simulink subsystem "US_016"  (R2023b)
settings: Solver=VariableStepAuto  StartTime=0.0  StopTime=10.0  RelTol=1e-3
libraries: arduinolib x2
settings Model: Creator=javie  LastModifiedBy=javie

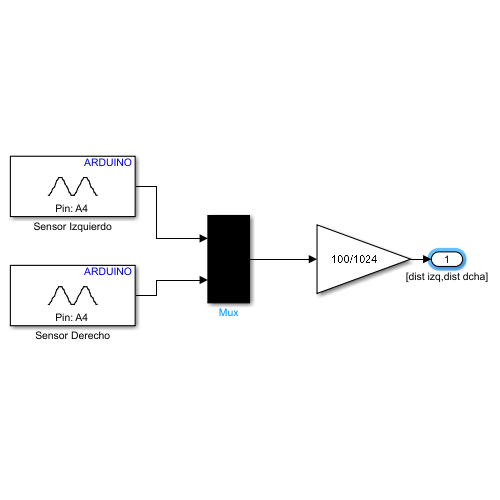
[thumbnail: Simulink's stored preview of the top-level diagram]
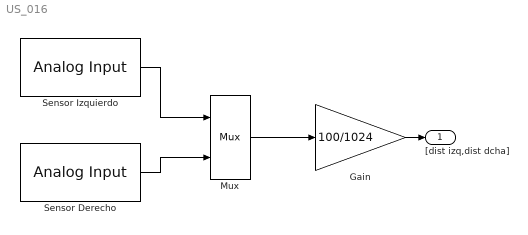
== system US_016 ==
  Gain : Gain  Gain=100/1024
  Mux : Mux  Inputs=2
  Sensor Derecho : arduinolib/Analog Input  pinNumber=4  ReadResultsOnly=off  ConversionTriggerSource=Software  ExternalTriggerType=uint32( 0 )  OutputDataType=uint16  EnableConversionCompleteNotify=off  EnableOuputStatus=off  SampleTime=-1  blockPlatform=arduino
  Sensor Izquierdo : arduinolib/Analog Input  pinNumber=4  ReadResultsOnly=off  ConversionTriggerSource=Software  ExternalTriggerType=uint32( 0 )  OutputDataType=uint16  EnableConversionCompleteNotify=off  EnableOuputStatus=off  SampleTime=-1  blockPlatform=arduino
  "[dist izq,dist dcha]" : Outport
  wires:
  Gain/1 -> "[dist izq,dist dcha]"/1
  Mux/1 -> Gain/1
  Sensor Derecho/1 -> Mux/2
  Sensor Izquierdo/1 -> Mux/1
